simulink model "ex1_Lab3_compatibil"  (R2018a)
settings: Solver=VariableStepAuto  StartTime=0.0  StopTime=50000.0  RelTol=1e-3
libraries: simulink x1
settings Model: Creator=Bogdi  LastModifiedBy=Bogdi
settings DataIOCC: ReturnWorkspaceOutputs=on
settings SFSimCC: SimUseLocalCustomCode=on
settings RTWCC: RTWUseLocalCustomCode=on

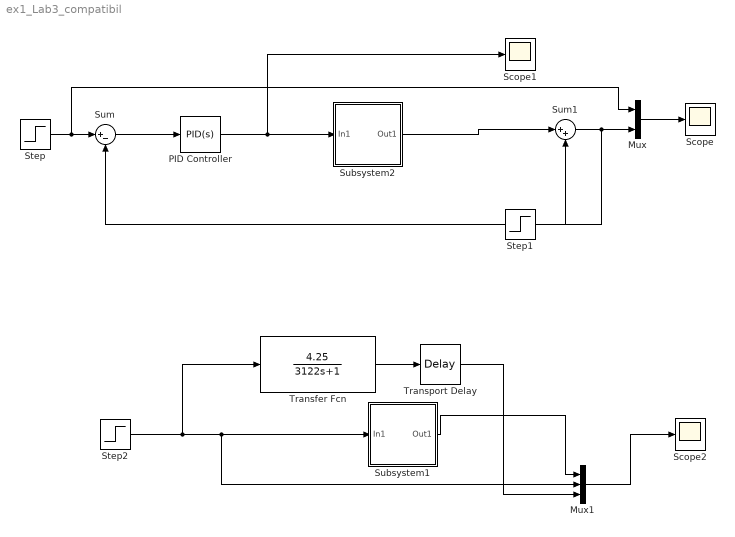
== system ex1_Lab3_compatibil ==
  Mux : Mux  Inputs=2
  Mux1 : Mux  Inputs=3
  PID Controller : simulink/Continuous/PID Controller  Controller=PID  Form=Parallel  TimeDomain=Continuous-time  SampleTime=-1  IntegratorMethod=Forward Euler  FilterMethod=Forward Euler  ControllerParametersSource=internal  P=1  I=1  D=0  UseFilter=on  N=100  TunerSelectOption=Transfer Function Based (PID Tuner App)  InitialConditionSource=internal  InitialConditionForIntegrator=0  InitialConditionForFilter=0  DifferentiatorICPrevScaledInput=0  ExternalReset=none  TrackingMode=off  Kt=1  LimitOutput=off  UpperSaturationLimit=inf  LowerSaturationLimit=-inf  LinearizeAsGain=on  AntiWindupMode=none  Kb=1  POutMin=[]  POutMax=[]  IOutMin=[]  IOutMax=[]  DOutMin=[]  DOutMax=[]  NOutMin=[]  NOutMax=[]  SumOutMin=[]  SumOutMax=[]  SaturationOutMin=[]  SaturationOutMax=[]  PParamMin=[]  PParamMax=[]  IParamMin=[]  IParamMax=[]  DParamMin=[]  DParamMax=[]  NParamMin=[]  NParamMax=[]  KbParamMin=[]  KbParamMax=[]  KtParamMin=[]  KtParamMax=[]  KbOutMin=[]  KbOutMax=[]  KtOutMin=[]  KtOutMax=[]  IntegratorOutMin=[]  IntegratorOutMax=[]  FilterOutMin=[]  FilterOutMax=[]  SumI1OutMin=[]  SumI1OutMax=[]  SumI2OutMin=[]  SumI2OutMax=[]  SumI3OutMin=[]  SumI3OutMax=[]  SumDOutMin=[]  SumDOutMax=[]  DifferentiatorOutMin=[]  DifferentiatorOutMax=[]  FilterDiffOutCoefMin=[]  FilterDiffOutCoefMax=[]  ReciprocalOutMin=[]  ReciprocalOutMax=[]  SumDenOutMin=[]  SumDenOutMax=[]  SumNumOutMin=[]  SumNumOutMax=[]  DivideOutMin=[]  DivideOutMax=[]  IntegratorContinuousStateAttributes=''  IntegratorStateMustResolveToSignalObject=off  IntegratorRTWStateStorageClass=Auto  FilterContinuousStateAttributes=''  FilterStateMustResolveToSignalObject=off  FilterRTWStateStorageClass=Auto
  Scope : Scope
  Scope1 : Scope
  Scope2 : Scope
  Step : Step  SampleTime=0
  Step1 : Step  SampleTime=0
  Step2 : Step  SampleTime=0
  Subsystem1 : Subsystem
  Subsystem2 : Subsystem
  Sum : Sum  Inputs=|+-
  Sum1 : Sum  Inputs=|++
  Transfer Fcn : TransferFcn  Numerator=[4.25]  Denominator="[3122  1 ]"
  Transport Delay : TransportDelay  DelayTime=941.4
  wires:
  Sum1/1 -> Sum/2, Mux/2
  Mux/1 -> Scope/1
  Sum/1 -> PID Controller/1
  PID Controller/1 -> Subsystem2/1(In1), Scope1/1
  Subsystem2/1(Out1) -> Sum1/1
  Step1/1 -> Sum1/2
  Step/1 -> Mux/1, Sum/1
  Step2/1 -> Transfer Fcn/1, Subsystem1/1(In1), Mux1/2
  Subsystem1/1(Out1) -> Mux1/1
  Mux1/1 -> Scope2/1
  Transfer Fcn/1 -> Transport Delay/1
  Transport Delay/1 -> Mux1/3

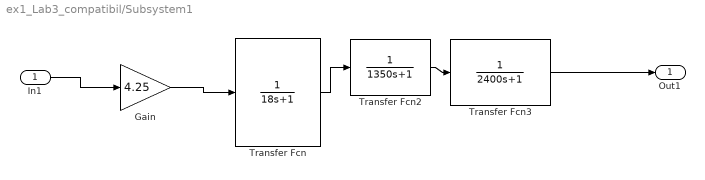
== system ex1_Lab3_compatibil/Subsystem1 ==
  In1 : Inport
  Gain : Gain  Gain=4.25
  Transfer Fcn : TransferFcn  Denominator=[18 1 ]
  Transfer Fcn2 : TransferFcn  Denominator=[1350 1]
  Transfer Fcn3 : TransferFcn  Denominator=[2400 1]
  Out1 : Outport
  wires:
  Gain/1 -> Transfer Fcn/1
  In1/1 -> Gain/1
  Transfer Fcn3/1 -> Out1/1
  Transfer Fcn/1 -> Transfer Fcn2/1
  Transfer Fcn2/1 -> Transfer Fcn3/1

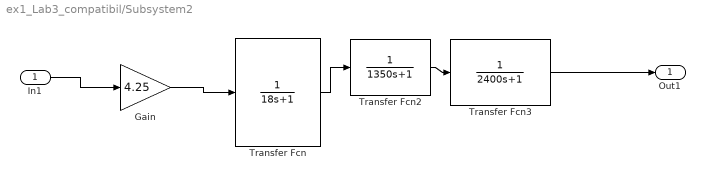
== system ex1_Lab3_compatibil/Subsystem2 ==
  In1 : Inport
  Gain : Gain  Gain=4.25
  Transfer Fcn : TransferFcn  Denominator=[18 1 ]
  Transfer Fcn2 : TransferFcn  Denominator=[1350 1]
  Transfer Fcn3 : TransferFcn  Denominator=[2400 1]
  Out1 : Outport
  wires:
  Gain/1 -> Transfer Fcn/1
  In1/1 -> Gain/1
  Transfer Fcn3/1 -> Out1/1
  Transfer Fcn/1 -> Transfer Fcn2/1
  Transfer Fcn2/1 -> Transfer Fcn3/1
